simulink model "BatteryManagementRing"  (R2020a)
settings: Solver=FixedStepDiscrete  StartTime=0.0  StopTime=10  FixedStep=Ts  RelTol=1e-3  EnableMultiTasking=on
undefined symbols (not defined in the file): BMR
libraries: simulink x4
settings Model: Creator=mukaipad  LastModifiedBy=Harjot
settings OptimizationCC: LifeSpan=inf
settings DebuggingCC: SFUnexpectedBacktrackingDiag=warning  SFNoUnconditionalDefaultTransitionDiag=warning  SFExecutionAtInitializationDiag=none  ArithmeticOperatorsInVariantConditions=warning
settings SFSimCC: SimUseLocalCustomCode=off  CustomCodeUndefinedFunction=UseInterfaceOnly
settings RTWCC: RTWUseLocalCustomCode=off
settings CodeAppCC: StateflowObjectComments=on
settings GRTTargetCC: TargetLangStandard=C89/C90 (ANSI)
settings ConfigComp: CovMetricSettings=dw  CovHtmlReporting=on  CovSaveCumulativeToWorkspaceVar=on  CovSaveSingleToWorkspaceVar=on  CovExternalEMLEnable=off

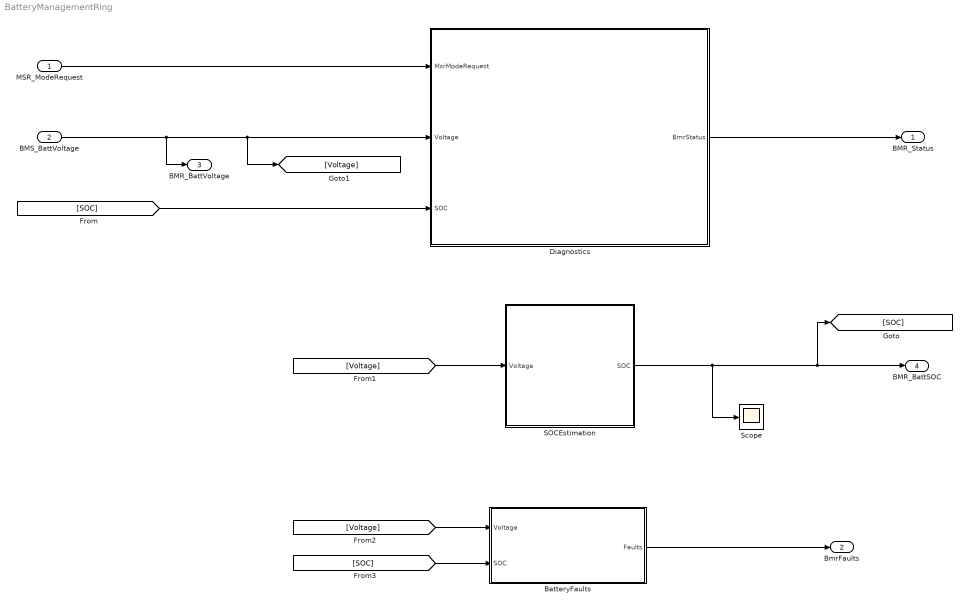
== system BatteryManagementRing ==
  MSR_ModeRequest : Inport
  BMS_BattVoltage : Inport  Port=2
  BatteryFaults : Subsystem
  Diagnostics : Stateflow chart  TreatAsAtomicUnit=on
  SOCEstimation : Subsystem
  Scope : Scope
  BMR_Status : Outport  VectorParamsAs1DForOutWhenUnconnected=off
  BmrFaults : Outport  Port=2  OutDataTypeStr=Bus: BatteryFaults  VectorParamsAs1DForOutWhenUnconnected=off
  BMR_BattVoltage : Outport  Port=3  VectorParamsAs1DForOutWhenUnconnected=off
  BMR_BattSOC : Outport  Port=4  VectorParamsAs1DForOutWhenUnconnected=off
  wires:
  [Voltage] -> BatteryFaults/1(Voltage)
  SOCEstimation/1(SOC) -> Scope/1, BMR_BattSOC/1, [SOC]
  [SOC] -> BatteryFaults/2(SOC)
  Diagnostics/1(BmrStatus) -> BMR_Status/1
  MSR_ModeRequest/1 -> Diagnostics/1(MsrModeRequest)
  [SOC] -> Diagnostics/3(SOC)
  [Voltage] -> SOCEstimation/1(Voltage)
  BMS_BattVoltage/1 -> BMR_BattVoltage/1, Diagnostics/2(Voltage), [Voltage]
  BatteryFaults/1(Faults) -> BmrFaults/1

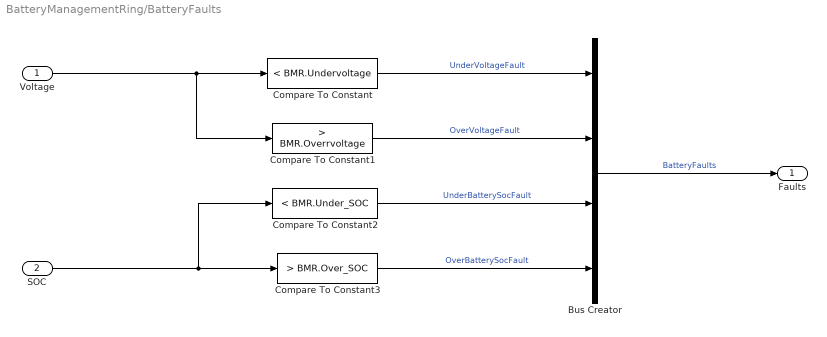
== system BatteryManagementRing/BatteryFaults ==
  Voltage : Inport
  SOC : Inport  Port=2
  Bus Creator : BusCreator  Inputs=4
  Compare To Constant : simulink/Logic and Bit Operations/Compare To Constant  relop=<  const=BMR.Undervoltage  OutDataTypeStr=boolean
  Compare To Constant1 : simulink/Logic and Bit Operations/Compare To Constant  relop=>  const=BMR.Overrvoltage  OutDataTypeStr=boolean
  Compare To Constant2 : simulink/Logic and Bit Operations/Compare To Constant  relop=<  const=BMR.Under_SOC  OutDataTypeStr=boolean
  Compare To Constant3 : simulink/Logic and Bit Operations/Compare To Constant  relop=>  const=BMR.Over_SOC  OutDataTypeStr=boolean
  Faults : Outport  VectorParamsAs1DForOutWhenUnconnected=off
  wires:
  Compare To Constant/1 -> Bus Creator/1  "UnderVoltageFault"
  Voltage/1 -> Compare To Constant1/1, Compare To Constant/1
  Compare To Constant1/1 -> Bus Creator/2  "OverVoltageFault"
  Compare To Constant2/1 -> Bus Creator/3  "UnderBatterySocFault"
  Compare To Constant3/1 -> Bus Creator/4  "OverBatterySocFault"
  SOC/1 -> Compare To Constant2/1, Compare To Constant3/1
  Bus Creator/1 -> Faults/1  "BatteryFaults"

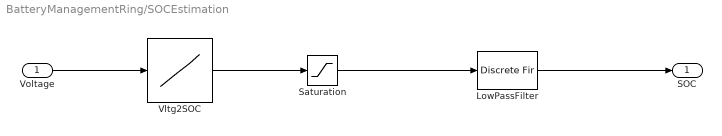
== system BatteryManagementRing/SOCEstimation ==
  Voltage : Inport
  LowPassFilter : DiscreteFir  Coefficients=[20:-1:0]/sum([20:-1:0])  SampleTime=0.001
  Saturation : Saturate  UpperLimit=1  LowerLimit=0
  Vltg2SOC : Lookup_n-D  NumberOfTableDimensions=1  BreakpointsForDimension1=BMR.Batt.SOC.Voltage  Table=BMR.Batt.SOC.SOC  InternalRulePriority=Speed  RndMeth=Simplest  InputSameDT=on
  SOC : Outport  VectorParamsAs1DForOutWhenUnconnected=off
  wires:
  Saturation/1 -> LowPassFilter/1
  Voltage/1 -> Vltg2SOC/1
  Vltg2SOC/1 -> Saturation/1
  LowPassFilter/1 -> SOC/1

== stateflow chart BatteryManagementRing/Diagnostics ==
  state SHUTDOWN
    entry:
    BmrStatus =  RING_STATUS.SHUTDOWN_COMPLETE_LV;
  state OFF
    entry:
    BmrStatus  =  RING_STATUS.OFF;
  state OPERATIONAL
    state RUNNING
      entry:
      BmrStatus =  RING_STATUS.RUNNING;
      state NORMAL_POWER
        entry:
      state RUNNING_POWERSAVE
        entry:
        %report low power
      (default) -> NORMAL_POWER
      NORMAL_POWER -> RUNNING_POWERSAVE : [Voltage < BMR.Running.MinVoltage &&  SOC < BMR.Running.MinSOC]
    state STARTUP
      entry:
      BmrStatus =  RING_STATUS.STARTUP_IN_PROGRESS_LV;
      % Test Voltage within range
      % Ensure sufficient voltage/SOC for startup
      state STARTUP_PASS
        entry:
        BmrStatus =  RING_STATUS.STARTUP_COMPLETE_LV;
      state STARTUP_INPROGRESS
      state STARTUP_LOWENERGY
        entry:
        %report low voltage battery error
      (default) -> STARTUP_INPROGRESS
      STARTUP_INPROGRESS -> STARTUP_PASS [order 2]
      STARTUP_INPROGRESS -> STARTUP_LOWENERGY [order 1] : [Voltage < BMR.Startup.MinVoltage ||  SOC < BMR.Startup.MinSOC && after(10,msec)]
    (default) -> STARTUP
    STARTUP -> RUNNING : [MsrModeRequest == MSR_REQUEST.RUNNING && BmrStatus == RING_STATUS.STARTUP_COMPLETE_LV]
  (default) -> OFF
  OFF -> OPERATIONAL : [MsrModeRequest == MSR_REQUEST.STARTUP_LV]
  OPERATIONAL -> SHUTDOWN : [MsrModeRequest == MSR_REQUEST.SHUTDOWN_LV]
  data: MsrModeRequest input Enum: MSR_REQUEST; Voltage input; SOC input; BmrStatus output Enum: RING_STATUS; BMR parameter
